simulink model "testDCL"  (R2022a)
settings: Solver=VariableStepAuto  StartTime=0.0  StopTime=Inf  MaxStep=1e-3  RelTol=1e-3
undefined symbols (not defined in the file): Call, Function, Neg, Pos
libraries: fl_lib x2, nesl_utility x2, ee_lib x2
settings Model: Creator=mmarq  LastModifiedBy=mmarq

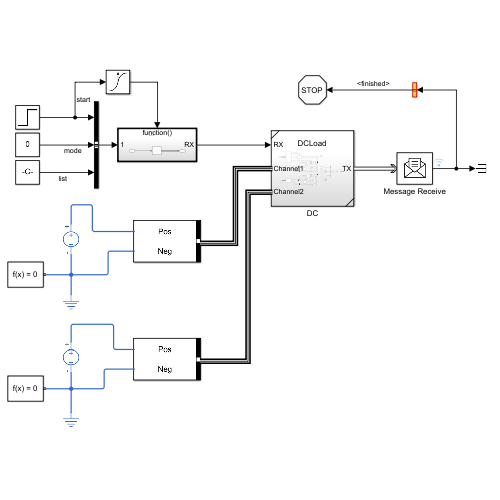
[thumbnail: Simulink's stored preview of the top-level diagram]
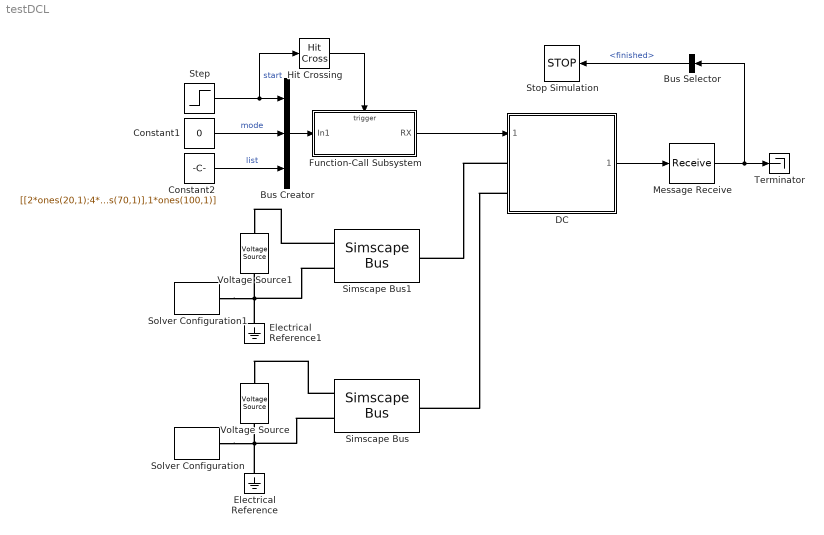
== system testDCL ==
  Bus Creator : BusCreator  Inputs=3  OutDataTypeStr=Bus: DCLCmd  NonVirtualBus=on
      settings: InheritFromInputs=off
  Bus Selector : BusSelector  OutputSignals=finished
  Constant1 : Constant  Value=0
  Constant2 : Constant  Value=[[2*ones(20,1);4*ones(10,1);10*ones(70,1)],1*ones(100,1)]
  DC : Subsystem  ReferencedSubsystem=DCLoad
  Electrical Reference : fl_lib/Electrical/Electrical Elements/Electrical Reference
      settings: SourceProductBaseCode=PW,SS,VE
  Electrical Reference1 : fl_lib/Electrical/Electrical Elements/Electrical Reference
      settings: SourceProductBaseCode=PW,SS,VE
  Function-Call Subsystem : Subsystem  TreatAsAtomicUnit=on
  Hit Crossing : HitCross  HitCrossingOffset=0.01  HitCrossingDirection=rising  HitCrossingOutputType=Function-Call
  Message Receive : Receive  InputPortMessageModes=m  ValueSourceWhenQueueIsEmpty=Use initial value
  Simscape Bus : SimscapeBus  HierarchyStrings=Pos;Neg
  Simscape Bus1 : SimscapeBus  HierarchyStrings=Pos;Neg
  Solver Configuration : nesl_utility/Solver Configuration  PhysicalDomain=network_engine_domain  SubClassName=solver  LeftPortType=input  RightPortType=generic  Tones=[]  Harmonics=[]  SimulateNoise=off  Profile=off  UseLocalSampling=off  EnableSwitchedLinearOptims=on  FrequencyDomain=off  UseCCode=off  RelTol=0.001  AbsTol=0.001  MinStep=1e-09  ToWorkspace=off  RevertToSquareIcSolve=off  NumHomotopyIterations=100  PhasorMode=off  PhasorModeNumHarmonics=1  IndexReductionMethod=DerivativeReplacement  DoDC=off  ResidualTolerance=1e-09  UseLocalSolver=off  LocalSolverChoice=NE_BACKWARD_EULER_ADVANCER  LocalSolverSampleTime=0.001  DoFixedCost=off  MaxNonlinIter=3  MaxModeIter=2  ComputeImpulses=off  ImpulseIterations=2  LinearAlgebra=auto  LinearAlgebraNumThread=0  EquationFormulation=NE_TIME_EF  DelaysMemoryBudget=1024  AutomaticFiltering=on  FilteringTimeConstant=0.001  PartitionStorageMethod=AS_NEEDED  PartitionMemoryBudget=1024  PartitionMethod=ROBUST
      settings: SourceProductBaseCode=SS,PW,VE
  Solver Configuration1 : nesl_utility/Solver Configuration  PhysicalDomain=network_engine_domain  SubClassName=solver  LeftPortType=input  RightPortType=generic  Tones=[]  Harmonics=[]  SimulateNoise=off  Profile=off  UseLocalSampling=off  EnableSwitchedLinearOptims=on  FrequencyDomain=off  UseCCode=off  RelTol=0.001  AbsTol=0.001  MinStep=1e-09  ToWorkspace=off  RevertToSquareIcSolve=off  NumHomotopyIterations=100  PhasorMode=off  PhasorModeNumHarmonics=1  IndexReductionMethod=DerivativeReplacement  DoDC=off  ResidualTolerance=1e-09  UseLocalSolver=off  LocalSolverChoice=NE_BACKWARD_EULER_ADVANCER  LocalSolverSampleTime=0.001  DoFixedCost=off  MaxNonlinIter=3  MaxModeIter=2  ComputeImpulses=off  ImpulseIterations=2  LinearAlgebra=auto  LinearAlgebraNumThread=0  EquationFormulation=NE_TIME_EF  DelaysMemoryBudget=1024  AutomaticFiltering=on  FilteringTimeConstant=0.001  PartitionStorageMethod=AS_NEEDED  PartitionMemoryBudget=1024  PartitionMethod=ROBUST
      settings: SourceProductBaseCode=SS,PW,VE
  Step : Step  SampleTime=0
  Stop Simulation : Stop
  Terminator : Terminator
  Voltage Source : ee_lib/Sources/Voltage Source  dc_voltage=15 V  ac_voltage=0 V  ac_shift=0 rad  ac_frequency=60 Hz  noise_mode=0  PSD=0 V^2/Hz  repeatability=1  auto_seed=3890346746  user_seed=0  sample_time=1e-3 s  i_specify=off  i_priority=None  i=0 A  i_nominal_specify=off  i_nominal_unit=A  i_nominal_value=1  v_specify=off  v_priority=None  v=0 V  v_nominal_specify=off  v_nominal_unit=V  v_nominal_value=1
  Voltage Source1 : ee_lib/Sources/Voltage Source  dc_voltage=15 V  ac_voltage=0 V  ac_shift=0 rad  ac_frequency=60 Hz  noise_mode=0  PSD=0 V^2/Hz  repeatability=1  auto_seed=545404223  user_seed=0  sample_time=1e-3 s  i_specify=off  i_priority=None  i=0 A  i_nominal_specify=off  i_nominal_unit=A  i_nominal_value=1  v_specify=off  v_priority=None  v=0 V  v_nominal_specify=off  v_nominal_unit=V  v_nominal_value=1
  wires:
  Step/1 -> Hit Crossing/1, Bus Creator/1  "start"
  Hit Crossing/1 -> Function-Call Subsystem/Trigger
  Bus Creator/1 -> Function-Call Subsystem/1(In1)
  Constant1/1 -> Bus Creator/2  "mode"
  Constant2/1 -> Bus Creator/3  "list"
  Function-Call Subsystem/1(RX) -> DC/1
  Bus Selector/1 -> Stop Simulation/1  "<finished>"
  DC/1 -> Message Receive/1
  Message Receive/1 -> Bus Selector/1, Terminator/1
  connections:
  Simscape Bus/LConn1 -- Voltage Source/LConn1
  Simscape Bus/LConn2 -- Electrical Reference/LConn1 -- Solver Configuration/RConn1 -- Voltage Source/RConn1
  DC/LConn2 -- Simscape Bus/RConn1
  Simscape Bus1/LConn2 -- Solver Configuration1/RConn1 -- Electrical Reference1/LConn1 -- Voltage Source1/RConn1
  Simscape Bus1/LConn1 -- Voltage Source1/LConn1
  DC/LConn1 -- Simscape Bus1/RConn1

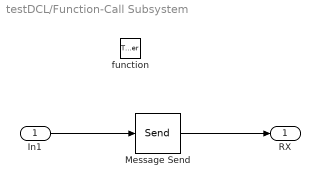
== system testDCL/Function-Call Subsystem ==
  In1 : Inport
  function : TriggerPort  TriggerType=function-call  VariantControl=(inherit)
  Message Send : Send  OutputPortMessageModes=m
  RX : Outport
  wires:
  In1/1 -> Message Send/1
  Message Send/1 -> RX/1
